simulink model "model"  (R2023b)
settings: Solver=FixedStepAuto  StartTime=0.0  StopTime=T_sim  FixedStep=delta_t  RelTol=1e-3
values from neighbouring files (symbols this model uses):
  alpha_ip = rand()    [main.m]
  alpha_pe = rand()    [main.m]
  alpha_pi = -rand()    [main.m]
  alpha_ps = rand()    [main.m]
  alpha_sp = rand()    [main.m]
  h_ip = 1    [main.m]
  h_pe = 1    [main.m]
  h_pi = 1    [main.m]
  h_ps = 1    [main.m]
  h_sp = 1    [main.m]
  lambda = 3    [main.m]
  tau_ip = rand()    [main.m]
  tau_pe = rand()    [main.m]
  tau_pi = rand()    [main.m]
  tau_ps = rand()    [main.m]
  tau_sp = rand()    [main.m]
settings Model: Creator=user  LastModifiedBy=user

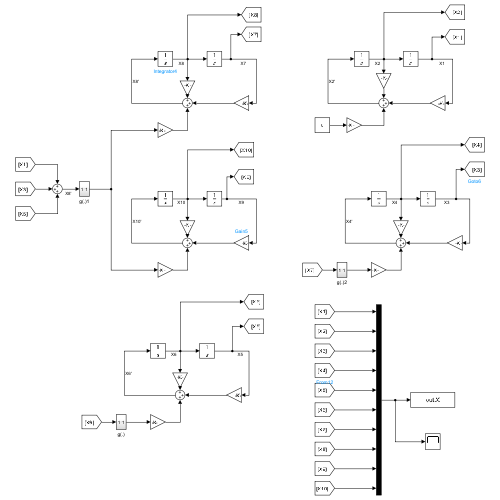
[thumbnail: Simulink's stored preview of the top-level diagram]
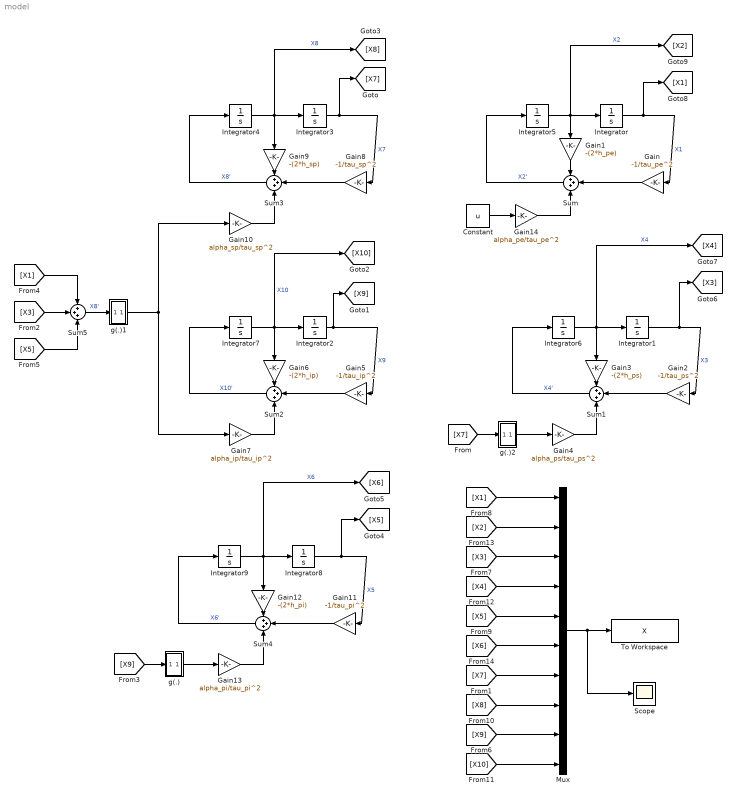
== system model ==
  Constant : Constant  Value=u  VectorParams1D=off
  Gain : Gain  Gain=-1/tau_pe^2
  Gain1 : Gain  Gain=-(2*h_pe)
  Gain10 : Gain  Gain=alpha_sp/tau_sp^2
  Gain11 : Gain  Gain=-1/tau_pi^2
  Gain12 : Gain  Gain=-(2*h_pi)
  Gain13 : Gain  Gain=alpha_pi/tau_pi^2
  Gain14 : Gain  Gain=alpha_pe/tau_pe^2
  Gain2 : Gain  Gain=-1/tau_ps^2
  Gain3 : Gain  Gain=-(2*h_ps)
  Gain4 : Gain  Gain=alpha_ps/tau_ps^2
  Gain5 : Gain  Gain=-1/tau_ip^2
  Gain6 : Gain  Gain=-(2*h_ip)
  Gain7 : Gain  Gain=alpha_ip/tau_ip^2
  Gain8 : Gain  Gain=-1/tau_sp^2
  Gain9 : Gain  Gain=-(2*h_sp)
  Integrator{,1..9} (10 alike) : Integrator
  Mux : Mux  Inputs=10
  Scope : Scope
  Sum{,1..5} (6 alike) : Sum  Inputs=+++
  To Workspace : ToWorkspace  VariableName=X  SampleTime=-1
  g(.) : Subsystem
  g(.)1 : Subsystem
  g(.)2 : Subsystem
  wires:
  Integrator5/1 -> [X2], Integrator/1, Gain1/1  "X2"
  Integrator/1 -> [X1], Gain/1  "X1"
  Gain/1 -> Sum/2
  Gain1/1 -> Sum/1
  Sum/1 -> Integrator5/1  "X2'"
  Gain2/1 -> Sum1/2
  Gain3/1 -> Sum1/1
  Integrator6/1 -> [X4], Integrator1/1, Gain3/1  "X4"
  Integrator1/1 -> [X3], Gain2/1  "X3"
  Sum1/1 -> Integrator6/1  "X4'"
  Gain4/1 -> Sum1/3
  [X7] -> g(.)2/1(In1)
  g(.)2/1(Out1) -> Gain4/1
  Gain7/1 -> Sum2/3
  Sum2/1 -> Integrator7/1  "X10'"
  Gain6/1 -> Sum2/1
  Integrator7/1 -> [X10], Integrator2/1, Gain6/1  "X10"
  Integrator2/1 -> [X9], Gain5/1  "X9"
  Gain5/1 -> Sum2/2
  g(.)/1(Out1) -> Gain13/1
  Gain11/1 -> Sum4/2
  [X9] -> g(.)/1(In1)
  Integrator8/1 -> [X5], Gain11/1  "X5"
  Gain13/1 -> Sum4/3
  Gain12/1 -> Sum4/1
  Integrator9/1 -> [X6], Integrator8/1, Gain12/1  "X6"
  Sum4/1 -> Integrator9/1  "X6'"
  [X3] -> Sum5/2
  [X5] -> Sum5/3
  [X1] -> Sum5/1
  Constant/1 -> Gain14/1
  Gain14/1 -> Sum/3
  [X1] -> Mux/1
  [X2] -> Mux/2
  [X3] -> Mux/3
  [X4] -> Mux/4
  [X5] -> Mux/5
  [X6] -> Mux/6
  [X7] -> Mux/7
  [X8] -> Mux/8
  [X9] -> Mux/9
  [X10] -> Mux/10
  Gain9/1 -> Sum3/1
  Integrator3/1 -> [X7], Gain8/1  "X7"
  Sum3/1 -> Integrator4/1  "X8'"
  g(.)1/1(Out1) -> Gain7/1, Gain10/1
  Integrator4/1 -> [X8], Integrator3/1, Gain9/1  "X8"
  Gain8/1 -> Sum3/2
  Gain10/1 -> Sum3/3
  Sum5/1 -> g(.)1/1(In1)  "X8'"
  Mux/1 -> Scope/1, To Workspace/1

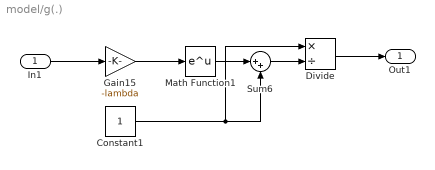
== system model/g(.) ==
  In1 : Inport
  Constant1 : Constant
  Divide : Product  Inputs=*/
  Gain15 : Gain  Gain=-lambda
  Math Function1 : Math
  Sum6 : Sum  Inputs=|++
  Out1 : Outport
  wires:
  Sum6/1 -> Divide/2
  Divide/1 -> Out1/1
  Math Function1/1 -> Sum6/1
  Constant1/1 -> Divide/1, Sum6/2
  In1/1 -> Gain15/1
  Gain15/1 -> Math Function1/1

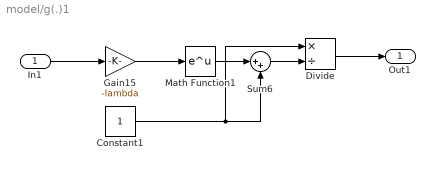
== system model/g(.)1 ==
  In1 : Inport
  Constant1 : Constant
  Divide : Product  Inputs=*/
  Gain15 : Gain  Gain=-lambda
  Math Function1 : Math
  Sum6 : Sum  Inputs=|++
  Out1 : Outport
  wires:
  Sum6/1 -> Divide/2
  Divide/1 -> Out1/1
  Math Function1/1 -> Sum6/1
  Constant1/1 -> Divide/1, Sum6/2
  In1/1 -> Gain15/1
  Gain15/1 -> Math Function1/1

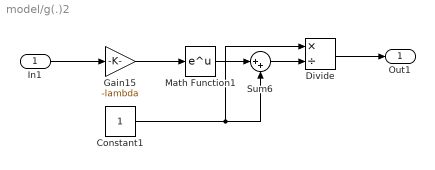
== system model/g(.)2 ==
  In1 : Inport
  Constant1 : Constant
  Divide : Product  Inputs=*/
  Gain15 : Gain  Gain=-lambda
  Math Function1 : Math
  Sum6 : Sum  Inputs=|++
  Out1 : Outport
  wires:
  Sum6/1 -> Divide/2
  Divide/1 -> Out1/1
  Math Function1/1 -> Sum6/1
  Constant1/1 -> Divide/1, Sum6/2
  In1/1 -> Gain15/1
  Gain15/1 -> Math Function1/1
